simulink model "BallAndPlateSimulation"  (R2019b)
settings: Solver=FixedStepAuto  StartTime=0.0  StopTime=t_experiment  FixedStep=0.001  RelTol=1e-3
values from neighbouring files (symbols this model uses):
  C_v = 16.5    [SimParameters.m]
  g = 9.81    [SimParameters.m]
  I_b = m_b*r_b^2    (= 8.664e-06)    [SimParameters.m]
  I_max = 3    [SimParameters.m]
  I_min = -3    [SimParameters.m]
  I_p = m_p*0.04^2/12    (= 0.00012)    [SimParameters.m]
  K = 11    [SimParameters.m]
  m_b = 0.024    [SimParameters.m]
  m_m = 0.118    [SimParameters.m]
  m_p = 0.9    [SimParameters.m]
  r = 0.17    [SimParameters.m]
  r_b = 0.019    [SimParameters.m]
  Tdelay_bob = 1*10^-9    (= 1e-09)    [SimParameters.m]
  Tdelay_mp = 1*10^-9    (= 1e-09)    [SimParameters.m]
  ts_camera = 1/30    (= 0.0333333333333)    [SimParameters.m]
  ts_mp = 1/1000    (= 0.001)    [SimParameters.m]
  Ybop0 = [0; 0; 0; 0]    [SimParameters.m]
  Ymp0 = [0; 0; 0; 0; 0; Zoffset]    [SimParameters.m]
  Zoffset = 0.32    [SimParameters.m]
undefined symbols (not defined in the file or in its folder): SimulateCamera, SimulateEncoders, SimulateTimeDelays, ts, UseNonlinearPlant
settings Model: Creator=Duintje  LastModifiedBy=chukh

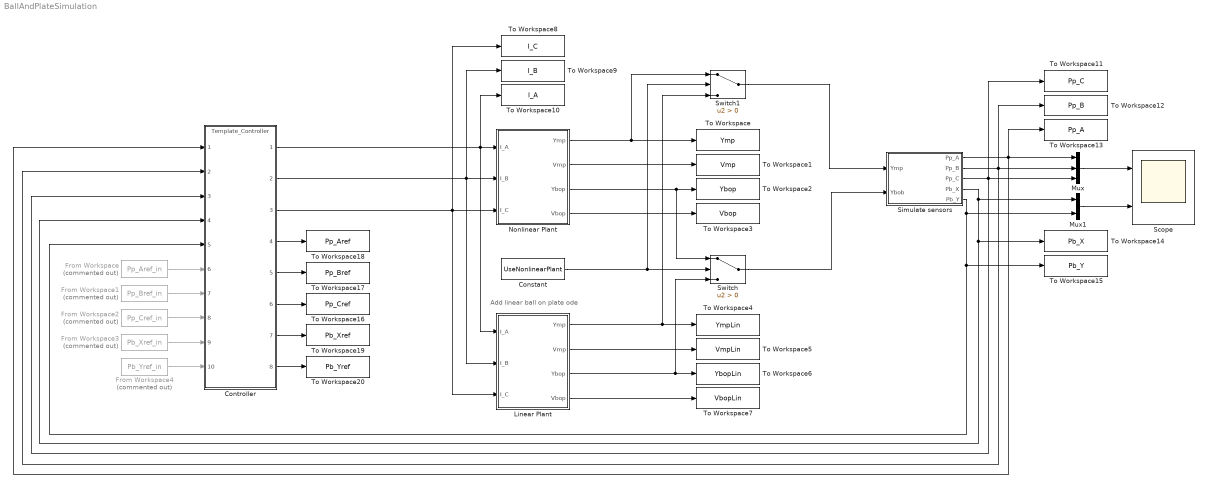
== system BallAndPlateSimulation ==
  note: Add linear ball on plate ode
  Constant : Constant  Value=UseNonlinearPlant
  Controller : ModelReference  ModelNameDialog=Template_Controller.slx  SimulationMode=Normal  ModelReferenceVersion=1.21
  From Workspace : FromWorkspace  Commented=on  VariableName=Pp_Aref_in  SampleTime=ts  Interpolate=off  OutputAfterFinalValue=Holding final value
  From Workspace1 : FromWorkspace  Commented=on  VariableName=Pp_Bref_in  SampleTime=ts  Interpolate=off  OutputAfterFinalValue=Holding final value
  From Workspace2 : FromWorkspace  Commented=on  VariableName=Pp_Cref_in  SampleTime=ts  Interpolate=off  OutputAfterFinalValue=Holding final value
  From Workspace3 : FromWorkspace  Commented=on  VariableName=Pb_Xref_in  SampleTime=ts  Interpolate=off  OutputAfterFinalValue=Holding final value
  From Workspace4 : FromWorkspace  Commented=on  VariableName=Pb_Yref_in  SampleTime=ts  Interpolate=off  OutputAfterFinalValue=Holding final value
  Linear Plant : Subsystem
  Mux : Mux  Inputs=3
  Mux1 : Mux  Inputs=2
  Nonlinear Plant : Subsystem
  Scope : Scope  NumInputPorts=2
  Simulate sensors : Subsystem
  Switch : Switch  Criteria=u2 > Threshold
  Switch1 : Switch  Criteria=u2 > Threshold
  To Workspace : ToWorkspace  VariableName=Ymp  SampleTime=-1
  To Workspace1 : ToWorkspace  VariableName=Vmp  SampleTime=-1
  To Workspace10 : ToWorkspace  VariableName=I_A  SampleTime=-1
  To Workspace11 : ToWorkspace  VariableName=Pp_C  SampleTime=-1
  To Workspace12 : ToWorkspace  VariableName=Pp_B  SampleTime=-1
  To Workspace13 : ToWorkspace  VariableName=Pp_A  SampleTime=-1
  To Workspace14 : ToWorkspace  VariableName=Pb_X  SampleTime=-1
  To Workspace15 : ToWorkspace  VariableName=Pb_Y  SampleTime=-1
  To Workspace16 : ToWorkspace  VariableName=Pp_Cref  SampleTime=-1
  To Workspace17 : ToWorkspace  VariableName=Pp_Bref  SampleTime=-1
  To Workspace18 : ToWorkspace  VariableName=Pp_Aref  SampleTime=-1
  To Workspace19 : ToWorkspace  VariableName=Pb_Xref  SampleTime=-1
  To Workspace2 : ToWorkspace  VariableName=Ybop  SampleTime=-1
  To Workspace20 : ToWorkspace  VariableName=Pb_Yref  SampleTime=-1
  To Workspace3 : ToWorkspace  VariableName=Vbop  SampleTime=-1
  To Workspace4 : ToWorkspace  VariableName=YmpLin  SampleTime=-1
  To Workspace5 : ToWorkspace  VariableName=VmpLin  SampleTime=-1
  To Workspace6 : ToWorkspace  VariableName=YbopLin  SampleTime=-1
  To Workspace7 : ToWorkspace  VariableName=VbopLin  SampleTime=-1
  To Workspace8 : ToWorkspace  VariableName=I_C  SampleTime=-1
  To Workspace9 : ToWorkspace  VariableName=I_B  SampleTime=-1
  wires:
  Controller/1 -> Linear Plant/1(I_A), To Workspace10/1, Nonlinear Plant/1(I_A)
  Controller/2 -> To Workspace9/1, Linear Plant/2(I_B), Nonlinear Plant/2(I_B)
  Controller/3 -> Linear Plant/3(I_C), To Workspace8/1, Nonlinear Plant/3(I_C)
  Linear Plant/1(Ymp) -> Switch1/3, To Workspace4/1
  Linear Plant/2(Vmp) -> To Workspace5/1
  Linear Plant/3(Ybop) -> Switch/3, To Workspace6/1
  Linear Plant/4(Vbop) -> To Workspace7/1
  Nonlinear Plant/3(Ybop) -> Switch/1, To Workspace2/1
  Nonlinear Plant/2(Vmp) -> To Workspace1/1
  Nonlinear Plant/1(Ymp) -> Switch1/1, To Workspace/1
  Nonlinear Plant/4(Vbop) -> To Workspace3/1
  Constant/1 -> Switch1/2, Switch/2
  Switch/1 -> Simulate sensors/2(Ybob)
  Switch1/1 -> Simulate sensors/1(Ymp)
  Simulate sensors/1(Pp_A) -> Controller/1, To Workspace13/1, Mux/1
  Simulate sensors/2(Pp_B) -> Controller/2, To Workspace12/1, Mux/2
  Simulate sensors/3(Pp_C) -> Controller/3, To Workspace11/1, Mux/3
  Mux/1 -> Scope/1
  Simulate sensors/4(Pb_X) -> Mux1/1, Controller/4, To Workspace14/1
  Simulate sensors/5(Pb_Y) -> Mux1/2, Controller/5, To Workspace15/1
  Mux1/1 -> Scope/2
  Controller/4 -> To Workspace18/1
  Controller/5 -> To Workspace17/1
  Controller/6 -> To Workspace16/1
  Controller/7 -> To Workspace19/1
  Controller/8 -> To Workspace20/1
  From Workspace4/1 -> Controller/10
  From Workspace3/1 -> Controller/9
  From Workspace2/1 -> Controller/8
  From Workspace1/1 -> Controller/7
  From Workspace/1 -> Controller/6

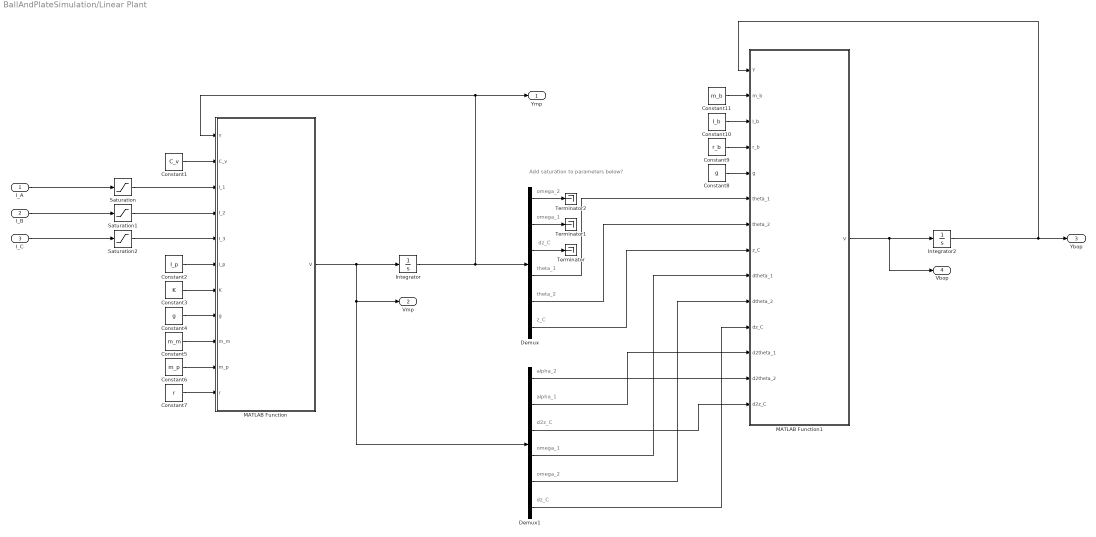
== system BallAndPlateSimulation/Linear Plant ==
  note: Add saturation to parameters below?
  note: omega_2
  note: omega_1
  note: dz_C
  note: theta_1
  note: theta_2
  note: z_C
  note: omega_1
  note: alpha_2
  note: omega_2
  note: alpha_1
  note: dz_C
  note: d2z_C
  I_A : Inport
  I_B : Inport  Port=2
  I_C : Inport  Port=3
  Constant1 : Constant  Value=C_v
  Constant10 : Constant  Value=I_b
  Constant11 : Constant  Value=m_b
  Constant2 : Constant  Value=I_p
  Constant3 : Constant  Value=K
  Constant4 : Constant  Value=g
  Constant5 : Constant  Value=m_m
  Constant6 : Constant  Value=m_p
  Constant7 : Constant  Value=r
  Constant8 : Constant  Value=g
  Constant9 : Constant  Value=r_b
  Demux : Demux  Outputs=6
  Demux1 : Demux  Outputs=6
  Integrator : Integrator  InitialCondition=Ymp0
  Integrator2 : Integrator  InitialCondition=Ybop0
  MATLAB Function : MATLAB Function  TreatAsAtomicUnit=on
  MATLAB Function1 : MATLAB Function  TreatAsAtomicUnit=on
  Saturation : Saturate  UpperLimit=I_max  LowerLimit=I_min
  Saturation1 : Saturate  UpperLimit=I_max  LowerLimit=I_min
  Saturation2 : Saturate  UpperLimit=I_max  LowerLimit=I_min
  Terminator : Terminator
  Terminator1 : Terminator
  Terminator2 : Terminator
  Ymp : Outport
  Vmp : Outport  Port=2
  Ybop : Outport  Port=3
  Vbop : Outport  Port=4
  wires:
  MATLAB Function/1(V) -> Vmp/1, Demux1/1, Integrator/1
  MATLAB Function1/1(V) -> Vbop/1, Integrator2/1
  I_A/1 -> Saturation/1
  Saturation/1 -> MATLAB Function/3(I_1)
  Saturation1/1 -> MATLAB Function/4(I_2)
  Saturation2/1 -> MATLAB Function/5(I_3)
  Constant1/1 -> MATLAB Function/2(C_v)
  Constant2/1 -> MATLAB Function/6(I_p)
  Constant3/1 -> MATLAB Function/7(K)
  Constant4/1 -> MATLAB Function/8(g)
  Constant5/1 -> MATLAB Function/9(m_m)
  Constant6/1 -> MATLAB Function/10(m_p)
  Constant7/1 -> MATLAB Function/11(r)
  Demux1/1 -> MATLAB Function1/13(d2theta_2)
  Demux1/2 -> MATLAB Function1/12(d2theta_1)
  Demux1/6 -> MATLAB Function1/11(dz_C)
  Demux1/3 -> MATLAB Function1/14(d2z_C)
  Demux/6 -> MATLAB Function1/8(z_C)
  Constant8/1 -> MATLAB Function1/5(g)
  Constant9/1 -> MATLAB Function1/4(r_b)
  Constant11/1 -> MATLAB Function1/2(m_b)
  Constant10/1 -> MATLAB Function1/3(I_b)
  Integrator2/1 -> Ybop/1, MATLAB Function1/1(Y)
  I_B/1 -> Saturation1/1
  I_C/1 -> Saturation2/1
  Demux1/4 -> MATLAB Function1/9(dtheta_1)
  Demux1/5 -> MATLAB Function1/10(dtheta_2)
  Demux/5 -> MATLAB Function1/7(theta_2)
  Demux/4 -> MATLAB Function1/6(theta_1)
  Integrator/1 -> Demux/1, Ymp/1, MATLAB Function/1(Y)
  Demux/3 -> Terminator/1
  Demux/2 -> Terminator1/1
  Demux/1 -> Terminator2/1

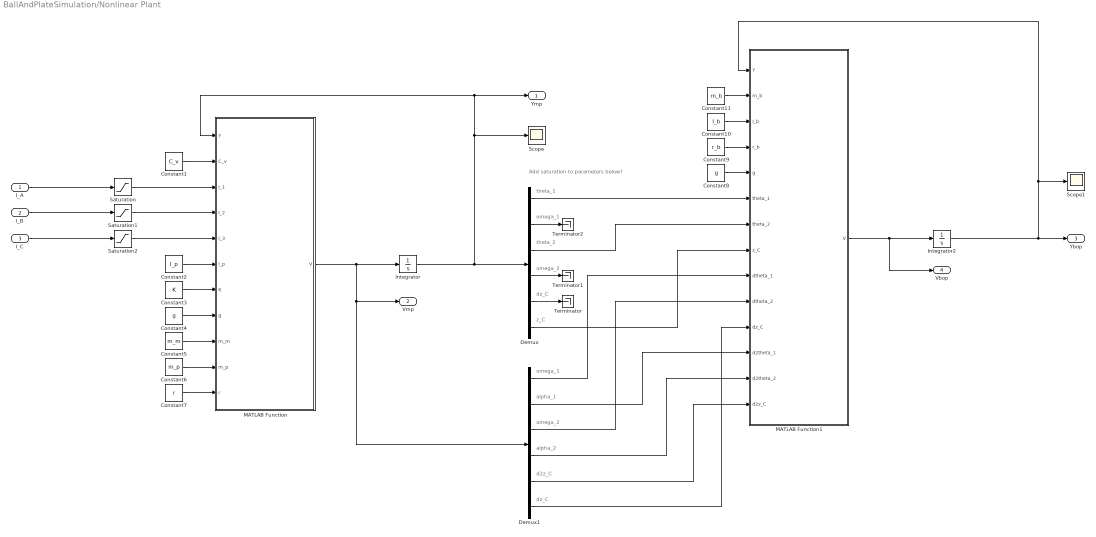
== system BallAndPlateSimulation/Nonlinear Plant ==
  note: Add saturation to parameters below?
  note: theta_1
  note: omega_1
  note: theta_2
  note: omega_2
  note: dz_C
  note: z_C
  note: alpha_2
  note: omega_1
  note: d2z_C
  note: alpha_1
  note: dz_C
  note: omega_2
  I_A : Inport
  I_B : Inport  Port=2
  I_C : Inport  Port=3
  Constant1 : Constant  Value=C_v
  Constant10 : Constant  Value=I_b
  Constant11 : Constant  Value=m_b
  Constant2 : Constant  Value=I_p
  Constant3 : Constant  Value=K
  Constant4 : Constant  Value=g
  Constant5 : Constant  Value=m_m
  Constant6 : Constant  Value=m_p
  Constant7 : Constant  Value=r
  Constant8 : Constant  Value=g
  Constant9 : Constant  Value=r_b
  Demux : Demux  Outputs=6
  Demux1 : Demux  Outputs=6
  Integrator : Integrator  InitialCondition=Ymp0
  Integrator2 : Integrator  InitialCondition=Ybop0
  MATLAB Function : MATLAB Function  TreatAsAtomicUnit=on
  MATLAB Function1 : MATLAB Function  TreatAsAtomicUnit=on
  Saturation : Saturate  UpperLimit=I_max  LowerLimit=I_min
  Saturation1 : Saturate  UpperLimit=I_max  LowerLimit=I_min
  Saturation2 : Saturate  UpperLimit=I_max  LowerLimit=I_min
  Scope : Scope
  Scope1 : Scope
  Terminator : Terminator
  Terminator1 : Terminator
  Terminator2 : Terminator
  Ymp : Outport
  Vmp : Outport  Port=2
  Ybop : Outport  Port=3
  Vbop : Outport  Port=4
  wires:
  MATLAB Function/1(V) -> Vmp/1, Demux1/1, Integrator/1
  MATLAB Function1/1(V) -> Vbop/1, Integrator2/1
  I_A/1 -> Saturation/1
  Saturation/1 -> MATLAB Function/3(I_1)
  Saturation1/1 -> MATLAB Function/4(I_2)
  Saturation2/1 -> MATLAB Function/5(I_3)
  Constant1/1 -> MATLAB Function/2(C_v)
  Constant2/1 -> MATLAB Function/6(I_p)
  Constant3/1 -> MATLAB Function/7(K)
  Constant4/1 -> MATLAB Function/8(g)
  Constant5/1 -> MATLAB Function/9(m_m)
  Constant6/1 -> MATLAB Function/10(m_p)
  Constant7/1 -> MATLAB Function/11(r)
  Integrator/1 -> Demux/1, Ymp/1, MATLAB Function/1(Y), Scope/1
  Demux/1 -> MATLAB Function1/6(theta_1)
  Demux1/1 -> MATLAB Function1/9(dtheta_1)
  Demux1/5 -> MATLAB Function1/14(d2z_C)
  Demux1/4 -> MATLAB Function1/13(d2theta_2)
  Demux1/2 -> MATLAB Function1/12(d2theta_1)
  Demux1/6 -> MATLAB Function1/11(dz_C)
  Demux1/3 -> MATLAB Function1/10(dtheta_2)
  Demux/6 -> MATLAB Function1/8(z_C)
  Demux/3 -> MATLAB Function1/7(theta_2)
  Constant8/1 -> MATLAB Function1/5(g)
  Constant9/1 -> MATLAB Function1/4(r_b)
  Constant11/1 -> MATLAB Function1/2(m_b)
  Constant10/1 -> MATLAB Function1/3(I_b)
  Integrator2/1 -> Ybop/1, Scope1/1, MATLAB Function1/1(Y)
  I_B/1 -> Saturation1/1
  I_C/1 -> Saturation2/1
  Demux/5 -> Terminator/1
  Demux/4 -> Terminator1/1
  Demux/2 -> Terminator2/1

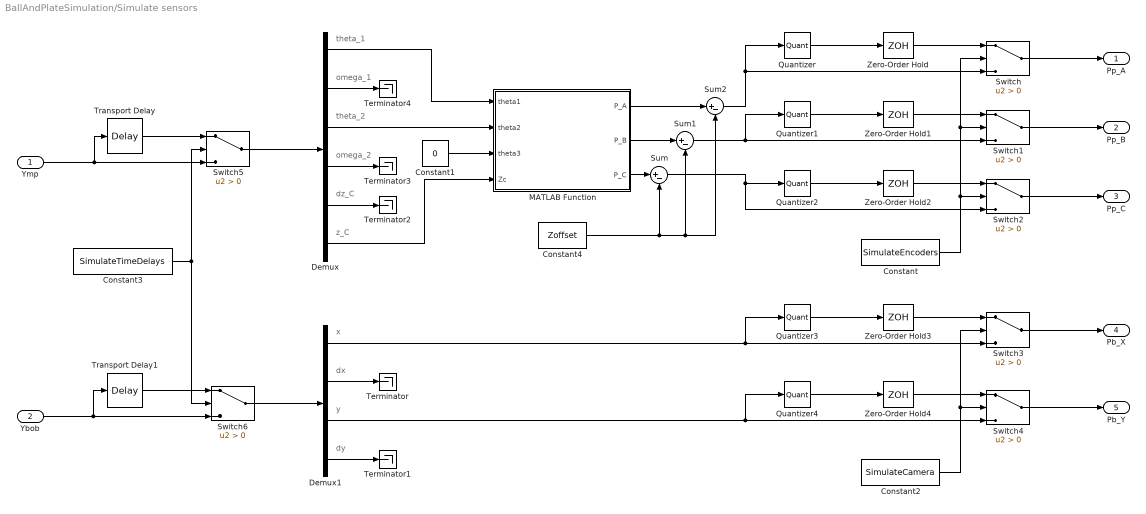
== system BallAndPlateSimulation/Simulate sensors ==
  note: dx
  note: dy
  note: x
  note: y
  note: theta_1
  note: omega_2
  note: dz_C
  note: theta_2
  note: z_C
  note: omega_1
  Ymp : Inport
  Ybob : Inport  Port=2
  Constant : Constant  Value=SimulateEncoders
  Constant1 : Constant  Value=0
  Constant2 : Constant  Value=SimulateCamera
  Constant3 : Constant  Value=SimulateTimeDelays
  Constant4 : Constant  Value=Zoffset
  Demux : Demux  Outputs=6
  Demux1 : Demux
  MATLAB Function : MATLAB Function  TreatAsAtomicUnit=on
  Quantizer : Quantizer  QuantizationInterval=EncStepSize
  Quantizer1 : Quantizer  QuantizationInterval=EncStepSize
  Quantizer2 : Quantizer  QuantizationInterval=EncStepSize
  Quantizer3 : Quantizer  QuantizationInterval=CameraStepSize
  Quantizer4 : Quantizer  QuantizationInterval=CameraStepSize
  Sum : Sum  Inputs=|+-
  Sum1 : Sum  Inputs=|+-
  Sum2 : Sum  Inputs=|+-
  Switch{,1..6} (7 alike) : Switch  Criteria=u2 > Threshold
  Terminator{,1..4} (5 alike) : Terminator
  Transport Delay : TransportDelay  DelayTime=Tdelay_mp
  Transport Delay1 : TransportDelay  DelayTime=Tdelay_bob
  Zero-Order Hold : ZeroOrderHold  SampleTime=ts_mp
  Zero-Order Hold1 : ZeroOrderHold  SampleTime=ts_mp
  Zero-Order Hold2 : ZeroOrderHold  SampleTime=ts_mp
  Zero-Order Hold3 : ZeroOrderHold  SampleTime=ts_camera
  Zero-Order Hold4 : ZeroOrderHold  SampleTime=ts_camera
  Pp_A : Outport
  Pp_B : Outport  Port=2
  Pp_C : Outport  Port=3
  Pb_X : Outport  Port=4
  Pb_Y : Outport  Port=5
  wires:
  Demux/3 -> MATLAB Function/2(theta2)
  Demux/6 -> MATLAB Function/4(Zc)
  Demux/1 -> MATLAB Function/1(theta1)
  Ymp/1 -> Transport Delay/1, Switch5/3
  Constant1/1 -> MATLAB Function/3(theta3)
  Sum2/1 -> Quantizer/1, Switch/3
  Zero-Order Hold/1 -> Switch/1
  Quantizer/1 -> Zero-Order Hold/1
  Switch/1 -> Pp_A/1
  Quantizer1/1 -> Zero-Order Hold1/1
  Switch1/1 -> Pp_B/1
  Zero-Order Hold1/1 -> Switch1/1
  Sum1/1 -> Quantizer1/1, Switch1/3
  Quantizer2/1 -> Zero-Order Hold2/1
  Switch2/1 -> Pp_C/1
  Zero-Order Hold2/1 -> Switch2/1
  Sum/1 -> Quantizer2/1, Switch2/3
  Constant/1 -> Switch2/2, Switch/2, Switch1/2
  Zero-Order Hold3/1 -> Switch3/1
  Quantizer3/1 -> Zero-Order Hold3/1
  Zero-Order Hold4/1 -> Switch4/1
  Demux1/3 -> Quantizer4/1, Switch4/3
  Constant2/1 -> Switch3/2, Switch4/2
  Switch4/1 -> Pb_Y/1
  Demux1/1 -> Quantizer3/1, Switch3/3
  Quantizer4/1 -> Zero-Order Hold4/1
  Switch3/1 -> Pb_X/1
  Switch5/1 -> Demux/1
  Transport Delay/1 -> Switch5/1
  Ybob/1 -> Switch6/3, Transport Delay1/1
  Switch6/1 -> Demux1/1
  Transport Delay1/1 -> Switch6/1
  Constant3/1 -> Switch5/2, Switch6/2
  MATLAB Function/3(P_C) -> Sum/1
  MATLAB Function/2(P_B) -> Sum1/1
  MATLAB Function/1(P_A) -> Sum2/1
  Constant4/1 -> Sum2/2, Sum1/2, Sum/2
  Demux1/2 -> Terminator/1
  Demux1/4 -> Terminator1/1
  Demux/5 -> Terminator2/1
  Demux/4 -> Terminator3/1
  Demux/2 -> Terminator4/1

== matlab function BallAndPlateSimulation/Nonlinear Plant/MATLAB Function1 ==
  data: Y input; V output; m_b input; I_b input; r_b input; g input; theta_1 input; theta_2 input; z_C input; dtheta_1 input; dtheta_2 input; dz_C input; d2theta_1 input; d2theta_2 input; d2z_C input
function V = ballOnPlateODE(Y,m_b,I_b,r_b,g,theta_1,theta_2,z_C,dtheta_1,dtheta_2,dz_C,d2theta_1,d2theta_2,d2z_C)
%BALLONPLATEODE
%    V = BALLONPLATEODE(Y,M_B,I_B,R_B,G,THETA_1,THETA_2,Z_C,DTHETA_1,DTHETA_2,DZ_C,D2THETA_1,D2THETA_2,D2Z_C)

%    This function was generated by the Symbolic Math Toolbox version 8.4.
%    26-May-2021 19:55:45

%matrix([[xf], [Dxf], [yf], [Dyf]])
t2 = cos(theta_1);
t3 = cos(theta_2);
t4 = sin(theta_1);
t5 = sin(theta_2);
t6 = Y(1);
t7 = Y(2);
t8 = Y(3);
t9 = Y(4);
t10 = dtheta_1.^2;
t11 = dtheta_2.^2;
t12 = r_b.^2;
t13 = r_b.^3;
t14 = t2.^2;
t15 = t2.^3;
t16 = t3.^2;
t18 = t3.^3;
t20 = t4.^2;
t21 = t4.^3;
t22 = t5.^2;
t24 = t5.^3;
t28 = m_b.*t12;
t17 = t14.^2;
t19 = t16.^2;
t23 = t20.^2;
t25 = t22.^2;
t26 = 1.0./t14;
t27 = 1.0./t16;
t29 = I_b+t28;
t30 = t14+t20;
t31 = 1.0./t29;
t32 = 1.0./t30;
V = [t7;(t26.*t27.*t31.*t32.*(I_b.*d2theta_2.*r_b.*t15.*t18+I_b.*r_b.*t11.*t15.*t24.*2.0-I_b.*t6.*t11.*t17.*t19-I_b.*t6.*t11.*t17.*t25.*2.0+d2z_C.*t5.*t17.*t18.*t28+g.*t5.*t17.*t18.*t28+m_b.*t11.*t13.*t15.*t24.*2.0-t6.*t11.*t17.*t25.*t28.*2.0+d2theta_2.*m_b.*t3.*t13.*t15.*t22+d2theta_1.*t5.*t8.*t16.*t17.*t28-d2theta_2.*t5.*t6.*t17.*t18.*t28-d2theta_2.*t3.*t6.*t17.*t24.*t28+dtheta_1.*t5.*t9.*t16.*t17.*t28.*2.0-dtheta_2.*t5.*t7.*t17.*t18.*t28.*2.0+dtheta_1.*t5.*t9.*t17.*t18.*t28-dtheta_2.*t3.*t7.*t17.*t24.*t28.*2.0+m_b.*t5.*t10.*t13.*t15.*t16.*2.0+m_b.*t5.*t11.*t13.*t15.*t16+t4.*t8.*t11.*t15.*t24.*t28.*2.0-t6.*t10.*t16.*t17.*t22.*t28-t6.*t11.*t16.*t17.*t22.*t28.*2.0+I_b.*dtheta_1.*dtheta_2.*r_b.*t18.*t21.*2.0+I_b.*dtheta_1.*dtheta_2.*t8.*t17.*t18.*2.0-I_b.*dtheta_1.*dtheta_2.*t8.*t17.*t19+I_b.*dtheta_1.*dtheta_2.*t8.*t18.*t23.*2.0+I_b.*d2theta_2.*r_b.*t2.*t18.*t20+I_b.*d2theta_2.*r_b.*t3.*t15.*t22+I_b.*d2theta_1.*t5.*t8.*t16.*t17+I_b.*d2theta_2.*t4.*t8.*t15.*t18-I_b.*d2theta_2.*t5.*t6.*t17.*t18-I_b.*d2theta_1.*t5.*t8.*t17.*t18+I_b.*d2theta_2.*t2.*t8.*t18.*t21-I_b.*d2theta_2.*t3.*t6.*t17.*t24+I_b.*dtheta_1.*t5.*t9.*t16.*t17.*2.0+I_b.*dtheta_2.*t4.*t9.*t15.*t18.*2.0-I_b.*dtheta_2.*t5.*t7.*t17.*t18.*2.0-I_b.*dtheta_1.*t5.*t9.*t17.*t18+I_b.*dtheta_2.*t2.*t9.*t18.*t21.*2.0-I_b.*dtheta_2.*t3.*t7.*t17.*t24.*2.0+I_b.*r_b.*t5.*t10.*t15.*t16+I_b.*r_b.*t5.*t11.*t15.*t16.*2.0+I_b.*r_b.*t2.*t11.*t20.*t24.*2.0+I_b.*t4.*t8.*t11.*t15.*t24.*2.0+I_b.*t2.*t8.*t11.*t21.*t24.*2.0-I_b.*t6.*t11.*t14.*t19.*t20-I_b.*t6.*t11.*t16.*t17.*t22.*3.0-I_b.*t6.*t11.*t14.*t20.*t25.*2.0+I_b.*dtheta_1.*dtheta_2.*r_b.*t4.*t14.*t18.*2.0-I_b.*dtheta_1.*dtheta_2.*r_b.*t4.*t14.*t22+I_b.*dtheta_1.*dtheta_2.*r_b.*t3.*t21.*t22.*2.0+I_b.*dtheta_1.*dtheta_2.*t4.*t6.*t15.*t24+I_b.*dtheta_1.*dtheta_2.*t3.*t8.*t17.*t22.*2.0+I_b.*dtheta_1.*dtheta_2.*t3.*t8.*t22.*t23.*2.0+I_b.*dtheta_1.*dtheta_2.*t8.*t14.*t18.*t20.*4.0-I_b.*dtheta_1.*dtheta_2.*t8.*t14.*t19.*t20-I_b.*dtheta_1.*dtheta_2.*t8.*t14.*t20.*t22-I_b.*d2theta_1.*r_b.*t3.*t4.*t5.*t14+I_b.*d2theta_1.*r_b.*t4.*t5.*t14.*t16+I_b.*d2theta_2.*r_b.*t2.*t3.*t20.*t22+I_b.*d2theta_1.*t3.*t4.*t6.*t15.*t22-I_b.*d2theta_1.*t3.*t5.*t8.*t14.*t20+I_b.*d2theta_2.*t3.*t4.*t8.*t15.*t22+I_b.*d2theta_2.*t2.*t3.*t8.*t21.*t22+I_b.*d2theta_1.*t5.*t8.*t14.*t16.*t20-I_b.*d2theta_2.*t5.*t6.*t14.*t18.*t20-I_b.*d2theta_2.*t3.*t6.*t14.*t20.*t24+I_b.*dtheta_1.*t3.*t4.*t7.*t15.*t22-I_b.*dtheta_1.*t3.*t5.*t9.*t14.*t20+I_b.*dtheta_2.*t3.*t4.*t9.*t15.*t22.*2.0+I_b.*dtheta_2.*t2.*t3.*t9.*t21.*t22.*2.0+I_b.*dtheta_1.*t5.*t9.*t14.*t16.*t20.*2.0-I_b.*dtheta_2.*t5.*t7.*t14.*t18.*t20.*2.0-I_b.*dtheta_2.*t3.*t7.*t14.*t20.*t24.*2.0+I_b.*r_b.*t2.*t5.*t10.*t16.*t20+I_b.*r_b.*t2.*t5.*t11.*t16.*t20.*2.0-I_b.*t3.*t4.*t5.*t8.*t10.*t15+I_b.*t4.*t5.*t8.*t10.*t15.*t16+I_b.*t4.*t5.*t8.*t11.*t15.*t16.*2.0+I_b.*t4.*t5.*t8.*t10.*t15.*t18+I_b.*t2.*t5.*t8.*t10.*t16.*t21+I_b.*t2.*t5.*t8.*t11.*t16.*t21.*2.0-I_b.*t3.*t6.*t10.*t14.*t20.*t22-I_b.*t6.*t11.*t14.*t16.*t20.*t22.*3.0+dtheta_1.*dtheta_2.*m_b.*t4.*t13.*t14.*t22-dtheta_1.*dtheta_2.*t4.*t6.*t15.*t24.*t28+dtheta_1.*dtheta_2.*t3.*t8.*t17.*t22.*t28.*2.0+dtheta_1.*dtheta_2.*t8.*t14.*t20.*t22.*t28+d2theta_1.*m_b.*t4.*t5.*t13.*t14.*t16+d2theta_2.*t3.*t4.*t8.*t15.*t22.*t28+d2theta_1.*t5.*t8.*t14.*t16.*t20.*t28-dtheta_1.*t3.*t4.*t7.*t15.*t22.*t28+dtheta_1.*t3.*t5.*t9.*t14.*t20.*t28+dtheta_2.*t3.*t4.*t9.*t15.*t22.*t28.*2.0+dtheta_1.*t5.*t9.*t14.*t16.*t20.*t28.*2.0+m_b.*t2.*t3.*t5.*t10.*t13.*t20.*2.0+m_b.*t2.*t5.*t10.*t13.*t16.*t20+t3.*t4.*t5.*t8.*t10.*t15.*t28+t2.*t3.*t5.*t8.*t10.*t21.*t28.*2.0+t4.*t5.*t8.*t10.*t15.*t16.*t28+t4.*t5.*t8.*t11.*t15.*t16.*t28+t4.*t5.*t8.*t10.*t15.*t18.*t28+t2.*t5.*t8.*t10.*t16.*t21.*t28-t3.*t6.*t10.*t14.*t20.*t22.*t28+I_b.*dtheta_1.*dtheta_2.*r_b.*t3.*t4.*t14.*t22.*2.0+I_b.*dtheta_1.*dtheta_2.*t4.*t5.*t6.*t15.*t16+I_b.*dtheta_1.*dtheta_2.*t3.*t8.*t14.*t20.*t22.*4.0-I_b.*dtheta_1.*dtheta_2.*t8.*t14.*t16.*t20.*t22+dtheta_1.*dtheta_2.*m_b.*t3.*t4.*t13.*t14.*t22.*2.0+dtheta_1.*dtheta_2.*t3.*t8.*t14.*t20.*t22.*t28.*2.0))./(t16+t22);t9;-t26.*t27.*t31.*t32.*(I_b.*d2theta_1.*r_b.*t3.*t15+I_b.*r_b.*t10.*t16.*t21.*2.0+I_b.*t3.*t8.*t10.*t17+I_b.*t8.*t10.*t16.*t17-I_b.*t8.*t10.*t17.*t18+I_b.*t8.*t10.*t16.*t23.*2.0+d2z_C.*t4.*t15.*t18.*t28+g.*t4.*t15.*t18.*t28+m_b.*t10.*t13.*t16.*t21.*2.0-t3.*t8.*t10.*t17.*t28+t8.*t10.*t16.*t17.*t28.*2.0-t8.*t10.*t17.*t18.*t28+t8.*t10.*t16.*t23.*t28.*2.0+d2theta_1.*m_b.*t2.*t13.*t16.*t20+d2theta_1.*t4.*t8.*t15.*t16.*t28-d2theta_2.*t4.*t6.*t15.*t18.*t28+d2theta_1.*t2.*t8.*t16.*t21.*t28-dtheta_1.*t3.*t4.*t9.*t15.*t28+dtheta_1.*t3.*t5.*t7.*t17.*t28+dtheta_1.*t4.*t9.*t15.*t16.*t28.*2.0-dtheta_2.*t4.*t7.*t15.*t18.*t28.*2.0+dtheta_1.*t4.*t9.*t15.*t18.*t28+dtheta_1.*t2.*t9.*t16.*t21.*t28.*2.0-m_b.*t3.*t4.*t10.*t13.*t14.*2.0+m_b.*t4.*t10.*t13.*t14.*t16.*3.0+m_b.*t4.*t11.*t13.*t14.*t16+m_b.*t4.*t11.*t13.*t14.*t22.*2.0-t3.*t8.*t10.*t14.*t20.*t28.*2.0-t4.*t6.*t11.*t15.*t24.*t28.*2.0+t8.*t10.*t14.*t16.*t20.*t28.*4.0+t8.*t11.*t14.*t16.*t20.*t28+t8.*t11.*t14.*t20.*t22.*t28.*2.0+I_b.*dtheta_1.*dtheta_2.*r_b.*t5.*t15-I_b.*dtheta_1.*dtheta_2.*t6.*t16.*t17-I_b.*dtheta_1.*dtheta_2.*t6.*t17.*t22+I_b.*d2theta_1.*r_b.*t2.*t16.*t20+I_b.*d2theta_1.*t3.*t4.*t8.*t15-I_b.*d2theta_1.*t3.*t5.*t6.*t17+I_b.*d2theta_1.*t4.*t8.*t15.*t16-I_b.*d2theta_1.*t4.*t8.*t15.*t18+I_b.*d2theta_1.*t2.*t8.*t16.*t21+I_b.*dtheta_1.*t3.*t4.*t9.*t15-I_b.*dtheta_1.*t3.*t5.*t7.*t17+I_b.*dtheta_1.*t4.*t9.*t15.*t16.*2.0-I_b.*dtheta_1.*t4.*t9.*t15.*t18+I_b.*dtheta_1.*t2.*t9.*t16.*t21.*2.0+I_b.*r_b.*t4.*t10.*t14.*t16.*2.0+I_b.*t8.*t10.*t14.*t16.*t20.*3.0-dtheta_1.*dtheta_2.*m_b.*t5.*t13.*t15+dtheta_1.*dtheta_2.*t6.*t17.*t22.*t28+I_b.*dtheta_1.*dtheta_2.*t4.*t5.*t8.*t15+I_b.*t3.*t4.*t5.*t6.*t10.*t15-dtheta_1.*dtheta_2.*t4.*t5.*t8.*t15.*t28+d2theta_2.*m_b.*t3.*t4.*t5.*t13.*t14-d2theta_2.*t3.*t4.*t6.*t15.*t22.*t28+d2theta_2.*t3.*t5.*t8.*t14.*t20.*t28-dtheta_2.*t3.*t4.*t7.*t15.*t22.*t28.*2.0+dtheta_2.*t3.*t5.*t9.*t14.*t20.*t28.*2.0+t3.*t4.*t5.*t6.*t10.*t15.*t28-t4.*t5.*t6.*t10.*t15.*t16.*t28-t4.*t5.*t6.*t11.*t15.*t16.*t28.*2.0+I_b.*dtheta_1.*dtheta_2.*t4.*t5.*t8.*t15.*t16+dtheta_1.*dtheta_2.*m_b.*t2.*t3.*t5.*t13.*t20.*2.0+dtheta_1.*dtheta_2.*t3.*t4.*t5.*t8.*t15.*t28.*2.0+dtheta_1.*dtheta_2.*t2.*t3.*t5.*t8.*t21.*t28.*2.0)];

== matlab function BallAndPlateSimulation/Nonlinear Plant/MATLAB Function ==
  data: Y input; V output; C_v input; I_1 input; I_2 input; I_3 input; I_p input; K input; g input; m_m input; m_p input; r input
function V = motorPlateODE(Y,C_v,I_1,I_2,I_3,I_p,K,g,m_m,m_p,r)
%MOTORPLATEODE
%    V = MOTORPLATEODE(Y,C_v,I_1,I_2,I_3,I_p,K,g,m_m,m_p,r)

%    This function was generated by the Symbolic Math Toolbox version 8.4.
%    18-May-2021 19:45:09

%matrix([[theta_1f], [omega_1f], [theta_2f], [omega_2f], [dz_Cf], [z_Cf]])
t2 = I_p.^2;
t3 = Y(1);
t4 = Y(2);
t5 = Y(3);
t6 = Y(4);
t7 = Y(5);
t8 = m_m.^2;
t9 = r.^2;
t10 = r.^3;
t19 = sqrt(3.0);
t11 = t9.^2;
t12 = cos(t3);
t13 = cos(t5);
t14 = sin(t3);
t15 = sin(t5);
t16 = t2.*4.0;
t17 = t4.^2;
t18 = t6.^2;
t20 = t12.^2;
t21 = t12.^3;
t22 = t13.^2;
t23 = t13.^3;
t25 = t14.^2;
t26 = t15.^2;
t24 = t22.^2;
t27 = I_p.*m_m.*t9.*t22.*6.0;
t29 = I_p.*m_m.*t9.*t25.*t26.*6.0;
t28 = t20.*t27;
t30 = t8.*t11.*t20.*t24.*9.0;
t31 = t16+t27+t28+t29+t30;
t32 = 1.0./t31;
V = [t4;t32.*(t12.*t14.*t17.*t27+t12.*t14.*t18.*t27+t8.*t11.*t12.*t14.*t17.*t24.*9.0+t8.*t11.*t12.*t14.*t18.*t24.*9.0-C_v.*I_p.*t4.*t9.*t20.*t22.*6.0-C_v.*m_m.*t4.*t11.*t20.*t24.*9.0+I_2.*I_p.*K.*r.*t12.*t13.*t19.*2.0-I_3.*I_p.*K.*r.*t12.*t13.*t19.*2.0+I_2.*K.*m_m.*t10.*t12.*t19.*t23.*3.0-I_3.*K.*m_m.*t10.*t12.*t19.*t23.*3.0+t4.*t6.*t8.*t11.*t15.*t20.*t23.*1.8e+1+t8.*t11.*t12.*t14.*t18.*t22.*t26.*1.8e+1-t8.*t11.*t14.*t18.*t21.*t22.*t26.*9.0-t8.*t11.*t12.*t14.^3.*t18.*t22.*t26.*9.0-t4.*t6.*t8.*t11.*t13.*t15.^3.*t20.*t25.*9.0+C_v.*I_p.*t6.*t9.*t12.*t13.*t14.*t15.*6.0-I_1.*K.*m_m.*t10.*t12.*t14.*t15.*t22.*6.0+I_2.*K.*m_m.*t10.*t12.*t14.*t15.*t22.*3.0+I_3.*K.*m_m.*t10.*t12.*t14.*t15.*t22.*3.0+I_p.*m_m.*t4.*t6.*t9.*t13.*t15.*t20.*1.2e+1+t4.*t6.*t8.*t11.*t13.*t15.*t20.*t25.*9.0-t4.*t6.*t8.*t11.*t15.*t20.*t23.*t25.*9.0);t6;-r.*t32.*(I_1.*I_p.*K.*t13.*4.0-I_2.*I_p.*K.*t13.*2.0-I_3.*I_p.*K.*t13.*2.0+C_v.*I_p.*r.*t6.*t22.*6.0-t8.*t10.*t15.*t18.*t20.*t23.*1.8e+1+t8.*t10.*t15.*t18.*t20.^2.*t23.*9.0+I_2.*I_p.*K.*t14.*t15.*t19.*2.0-I_3.*I_p.*K.*t14.*t15.*t19.*2.0+C_v.*I_p.*r.*t6.*t25.*t26.*6.0+I_1.*K.*m_m.*t9.*t20.*t23.*6.0-I_2.*K.*m_m.*t9.*t20.*t23.*3.0-I_3.*K.*m_m.*t9.*t20.*t23.*3.0+C_v.*m_m.*t6.*t10.*t20.*t24.*9.0-I_p.*m_m.*r.*t13.*t15.*t18.*1.2e+1-I_p.*m_m.*r.*t4.*t6.*t12.*t14.*6.0+I_p.*m_m.*r.*t13.*t15.*t18.*t20.*6.0+I_p.*m_m.*r.*t13.*t15.*t17.*t25.*6.0+I_p.*m_m.*r.*t13.*t15.*t18.*t25.*1.2e+1-t4.*t6.*t8.*t10.*t14.*t21.*t22.*9.0+t4.*t6.*t8.*t10.*t14.*t21.*t24.*9.0+t8.*t10.*t15.*t18.*t20.*t23.*t25.*9.0-C_v.*I_p.*r.*t4.*t12.*t13.*t14.*t15.*6.0+I_p.*m_m.*r.*t4.*t6.*t12.*t14.*t22.*6.0+I_p.*m_m.*r.*t4.*t6.*t12.*t14.*t26.*1.8e+1+t4.*t6.*t8.*t10.*t14.*t21.*t22.*t26.*9.0);-(C_v.*t7.*3.0+g.*m_m.*3.0+g.*m_p-I_1.*K-I_2.*K-I_3.*K)./(m_m.*3.0+m_p);t7];
end

== matlab function BallAndPlateSimulation/Linear Plant/MATLAB Function ==
  data: Y input; V output; C_v input; I_1 input; I_2 input; I_3 input; I_p input; K input; g input; m_m input; m_p input; r input
function V = motorPlateODElinear(Y,C_v,I_1,I_2,I_3,I_p,K,g,m_m,m_p,r)
%MOTORPLATEODELINEAR
%    V = MOTORPLATEODELINEAR(Y,C_v,I_1,I_2,I_3,I_p,K,g,m_m,m_p,r)

%    This function was generated by the Symbolic Math Toolbox version 58.4.
%    13-May-2021 20:04:38

%matrix([[omega_2f], [omega_1f], [dz_Cf], [theta_1f], [theta_2f], [z_Cf]])
t2 = I_p.*2.0;
t3 = Y(1);
t4 = Y(2);
t5 = Y(3);
t6 = r.^2;
t7 = I_2.*K;
t8 = I_3.*K;
t9 = sqrt(3.0);
t10 = -t7;
t11 = -t8;
t12 = m_m.*t6.*3.0;
t13 = t2+t12;
t14 = 1.0./t13;
V = [r.*t14.*(t7+t8-I_1.*K.*2.0-C_v.*r.*t3.*3.0);-r.*t14.*(t8.*t9+t9.*t10+C_v.*r.*t4.*3.0);-(m_p+t10+t11+C_v.*t5.*3.0+g.*m_m.*3.0-I_1.*K)./(m_m.*3.0+m_p);t4;t3;t5];
end

== matlab function BallAndPlateSimulation/Linear Plant/MATLAB Function1 ==
  data: Y input; V output; m_b input; I_b input; r_b input; g input; theta_1 input; theta_2 input; z_C input; dtheta_1 input; dtheta_2 input; dz_C input; d2theta_1 input; d2theta_2 input; d2z_C input
function V = ballOnPlateODE(Y,m_b,I_b,r_b,g,theta_1,theta_2,z_C,dtheta_1,dtheta_2,dz_C,d2theta_1,d2theta_2,d2z_C)
%BALLONPLATEODE
%    V = BALLONPLATEODE(Y,m_b,I_b,r_b,g,theta_1,theta_2,z_C,dtheta_1,dtheta_2,dz_C,d2theta_1,d2theta_2,d2z_C)

%    This function was generated by the Symbolic Math Toolbox version 8.4.
%    16-May-2021 00:03:52

%matrix([[xf], [Dxf], [yf], [Dyf]])
t2 = cos(theta_1);
t3 = cos(theta_2);
t4 = sin(theta_1);
t5 = sin(theta_2);
t6 = Y(1);
t7 = Y(2);
t8 = Y(3);
t9 = Y(4);
t10 = dtheta_1.^2;
t11 = dtheta_2.^2;
t12 = r_b.^2;
t13 = r_b.^3;
t14 = t2.^2;
t15 = t2.^3;
t16 = t3.^2;
t18 = t3.^3;
t20 = t4.^2;
t21 = t4.^3;
t22 = t5.^2;
t24 = t5.^3;
t28 = m_b.*t12;
t17 = t14.^2;
t19 = t16.^2;
t23 = t20.^2;
t25 = t22.^2;
t26 = 1.0./t14;
t27 = 1.0./t16;
t29 = I_b+t28;
t30 = t14+t20;
t31 = 1.0./t29;
t32 = 1.0./t30;
V = [t7;(t26.*t27.*t31.*t32.*(I_b.*d2theta_2.*r_b.*t15.*t18+I_b.*r_b.*t11.*t15.*t24.*2.0-I_b.*t6.*t11.*t17.*t19-I_b.*t6.*t11.*t17.*t25.*2.0+d2z_C.*t5.*t17.*t18.*t28+g.*t5.*t17.*t18.*t28+m_b.*t11.*t13.*t15.*t24.*2.0-t6.*t11.*t17.*t25.*t28.*2.0+d2theta_2.*m_b.*t3.*t13.*t15.*t22+d2theta_1.*t5.*t8.*t16.*t17.*t28-d2theta_2.*t5.*t6.*t17.*t18.*t28-d2theta_2.*t3.*t6.*t17.*t24.*t28+dtheta_1.*t5.*t9.*t16.*t17.*t28.*2.0-dtheta_2.*t5.*t7.*t17.*t18.*t28.*2.0+dtheta_1.*t5.*t9.*t17.*t18.*t28-dtheta_2.*t3.*t7.*t17.*t24.*t28.*2.0+m_b.*t5.*t10.*t13.*t15.*t16.*2.0+m_b.*t5.*t11.*t13.*t15.*t16+t4.*t8.*t11.*t15.*t24.*t28.*2.0-t6.*t10.*t16.*t17.*t22.*t28-t6.*t11.*t16.*t17.*t22.*t28.*2.0+I_b.*dtheta_1.*dtheta_2.*r_b.*t18.*t21.*2.0+I_b.*dtheta_1.*dtheta_2.*t8.*t17.*t18.*2.0-I_b.*dtheta_1.*dtheta_2.*t8.*t17.*t19+I_b.*dtheta_1.*dtheta_2.*t8.*t18.*t23.*2.0+I_b.*d2theta_2.*r_b.*t2.*t18.*t20+I_b.*d2theta_2.*r_b.*t3.*t15.*t22+I_b.*d2theta_1.*t5.*t8.*t16.*t17+I_b.*d2theta_2.*t4.*t8.*t15.*t18-I_b.*d2theta_2.*t5.*t6.*t17.*t18-I_b.*d2theta_1.*t5.*t8.*t17.*t18+I_b.*d2theta_2.*t2.*t8.*t18.*t21-I_b.*d2theta_2.*t3.*t6.*t17.*t24+I_b.*dtheta_1.*t5.*t9.*t16.*t17.*2.0+I_b.*dtheta_2.*t4.*t9.*t15.*t18.*2.0-I_b.*dtheta_2.*t5.*t7.*t17.*t18.*2.0-I_b.*dtheta_1.*t5.*t9.*t17.*t18+I_b.*dtheta_2.*t2.*t9.*t18.*t21.*2.0-I_b.*dtheta_2.*t3.*t7.*t17.*t24.*2.0+I_b.*r_b.*t5.*t10.*t15.*t16+I_b.*r_b.*t5.*t11.*t15.*t16.*2.0+I_b.*r_b.*t2.*t11.*t20.*t24.*2.0+I_b.*t4.*t8.*t11.*t15.*t24.*2.0+I_b.*t2.*t8.*t11.*t21.*t24.*2.0-I_b.*t6.*t11.*t14.*t19.*t20-I_b.*t6.*t11.*t16.*t17.*t22.*3.0-I_b.*t6.*t11.*t14.*t20.*t25.*2.0+I_b.*dtheta_1.*dtheta_2.*r_b.*t4.*t14.*t18.*2.0-I_b.*dtheta_1.*dtheta_2.*r_b.*t4.*t14.*t22+I_b.*dtheta_1.*dtheta_2.*r_b.*t3.*t21.*t22.*2.0+I_b.*dtheta_1.*dtheta_2.*t4.*t6.*t15.*t24+I_b.*dtheta_1.*dtheta_2.*t3.*t8.*t17.*t22.*2.0+I_b.*dtheta_1.*dtheta_2.*t3.*t8.*t22.*t23.*2.0+I_b.*dtheta_1.*dtheta_2.*t8.*t14.*t18.*t20.*4.0-I_b.*dtheta_1.*dtheta_2.*t8.*t14.*t19.*t20-I_b.*dtheta_1.*dtheta_2.*t8.*t14.*t20.*t22-I_b.*d2theta_1.*r_b.*t3.*t4.*t5.*t14+I_b.*d2theta_1.*r_b.*t4.*t5.*t14.*t16+I_b.*d2theta_2.*r_b.*t2.*t3.*t20.*t22+I_b.*d2theta_1.*t3.*t4.*t6.*t15.*t22-I_b.*d2theta_1.*t3.*t5.*t8.*t14.*t20+I_b.*d2theta_2.*t3.*t4.*t8.*t15.*t22+I_b.*d2theta_2.*t2.*t3.*t8.*t21.*t22+I_b.*d2theta_1.*t5.*t8.*t14.*t16.*t20-I_b.*d2theta_2.*t5.*t6.*t14.*t18.*t20-I_b.*d2theta_2.*t3.*t6.*t14.*t20.*t24+I_b.*dtheta_1.*t3.*t4.*t7.*t15.*t22-I_b.*dtheta_1.*t3.*t5.*t9.*t14.*t20+I_b.*dtheta_2.*t3.*t4.*t9.*t15.*t22.*2.0+I_b.*dtheta_2.*t2.*t3.*t9.*t21.*t22.*2.0+I_b.*dtheta_1.*t5.*t9.*t14.*t16.*t20.*2.0-I_b.*dtheta_2.*t5.*t7.*t14.*t18.*t20.*2.0-I_b.*dtheta_2.*t3.*t7.*t14.*t20.*t24.*2.0+I_b.*r_b.*t2.*t5.*t10.*t16.*t20+I_b.*r_b.*t2.*t5.*t11.*t16.*t20.*2.0-I_b.*t3.*t4.*t5.*t8.*t10.*t15+I_b.*t4.*t5.*t8.*t10.*t15.*t16+I_b.*t4.*t5.*t8.*t11.*t15.*t16.*2.0+I_b.*t4.*t5.*t8.*t10.*t15.*t18+I_b.*t2.*t5.*t8.*t10.*t16.*t21+I_b.*t2.*t5.*t8.*t11.*t16.*t21.*2.0-I_b.*t3.*t6.*t10.*t14.*t20.*t22-I_b.*t6.*t11.*t14.*t16.*t20.*t22.*3.0+dtheta_1.*dtheta_2.*m_b.*t4.*t13.*t14.*t22-dtheta_1.*dtheta_2.*t4.*t6.*t15.*t24.*t28+dtheta_1.*dtheta_2.*t3.*t8.*t17.*t22.*t28.*2.0+dtheta_1.*dtheta_2.*t8.*t14.*t20.*t22.*t28+d2theta_1.*m_b.*t4.*t5.*t13.*t14.*t16+d2theta_2.*t3.*t4.*t8.*t15.*t22.*t28+d2theta_1.*t5.*t8.*t14.*t16.*t20.*t28-dtheta_1.*t3.*t4.*t7.*t15.*t22.*t28+dtheta_1.*t3.*t5.*t9.*t14.*t20.*t28+dtheta_2.*t3.*t4.*t9.*t15.*t22.*t28.*2.0+dtheta_1.*t5.*t9.*t14.*t16.*t20.*t28.*2.0+m_b.*t2.*t3.*t5.*t10.*t13.*t20.*2.0+m_b.*t2.*t5.*t10.*t13.*t16.*t20+t3.*t4.*t5.*t8.*t10.*t15.*t28+t2.*t3.*t5.*t8.*t10.*t21.*t28.*2.0+t4.*t5.*t8.*t10.*t15.*t16.*t28+t4.*t5.*t8.*t11.*t15.*t16.*t28+t4.*t5.*t8.*t10.*t15.*t18.*t28+t2.*t5.*t8.*t10.*t16.*t21.*t28-t3.*t6.*t10.*t14.*t20.*t22.*t28+I_b.*dtheta_1.*dtheta_2.*r_b.*t3.*t4.*t14.*t22.*2.0+I_b.*dtheta_1.*dtheta_2.*t4.*t5.*t6.*t15.*t16+I_b.*dtheta_1.*dtheta_2.*t3.*t8.*t14.*t20.*t22.*4.0-I_b.*dtheta_1.*dtheta_2.*t8.*t14.*t16.*t20.*t22+dtheta_1.*dtheta_2.*m_b.*t3.*t4.*t13.*t14.*t22.*2.0+dtheta_1.*dtheta_2.*t3.*t8.*t14.*t20.*t22.*t28.*2.0))./(t16+t22);t9;-t26.*t27.*t31.*t32.*(I_b.*d2theta_1.*r_b.*t3.*t15+I_b.*r_b.*t10.*t16.*t21.*2.0+I_b.*t3.*t8.*t10.*t17+I_b.*t8.*t10.*t16.*t17-I_b.*t8.*t10.*t17.*t18+I_b.*t8.*t10.*t16.*t23.*2.0+d2z_C.*t4.*t15.*t18.*t28+g.*t4.*t15.*t18.*t28+m_b.*t10.*t13.*t16.*t21.*2.0-t3.*t8.*t10.*t17.*t28+t8.*t10.*t16.*t17.*t28.*2.0-t8.*t10.*t17.*t18.*t28+t8.*t10.*t16.*t23.*t28.*2.0+d2theta_1.*m_b.*t2.*t13.*t16.*t20+d2theta_1.*t4.*t8.*t15.*t16.*t28-d2theta_2.*t4.*t6.*t15.*t18.*t28+d2theta_1.*t2.*t8.*t16.*t21.*t28-dtheta_1.*t3.*t4.*t9.*t15.*t28+dtheta_1.*t3.*t5.*t7.*t17.*t28+dtheta_1.*t4.*t9.*t15.*t16.*t28.*2.0-dtheta_2.*t4.*t7.*t15.*t18.*t28.*2.0+dtheta_1.*t4.*t9.*t15.*t18.*t28+dtheta_1.*t2.*t9.*t16.*t21.*t28.*2.0-m_b.*t3.*t4.*t10.*t13.*t14.*2.0+m_b.*t4.*t10.*t13.*t14.*t16.*3.0+m_b.*t4.*t11.*t13.*t14.*t16+m_b.*t4.*t11.*t13.*t14.*t22.*2.0-t3.*t8.*t10.*t14.*t20.*t28.*2.0-t4.*t6.*t11.*t15.*t24.*t28.*2.0+t8.*t10.*t14.*t16.*t20.*t28.*4.0+t8.*t11.*t14.*t16.*t20.*t28+t8.*t11.*t14.*t20.*t22.*t28.*2.0+I_b.*dtheta_1.*dtheta_2.*r_b.*t5.*t15-I_b.*dtheta_1.*dtheta_2.*t6.*t16.*t17-I_b.*dtheta_1.*dtheta_2.*t6.*t17.*t22+I_b.*d2theta_1.*r_b.*t2.*t16.*t20+I_b.*d2theta_1.*t3.*t4.*t8.*t15-I_b.*d2theta_1.*t3.*t5.*t6.*t17+I_b.*d2theta_1.*t4.*t8.*t15.*t16-I_b.*d2theta_1.*t4.*t8.*t15.*t18+I_b.*d2theta_1.*t2.*t8.*t16.*t21+I_b.*dtheta_1.*t3.*t4.*t9.*t15-I_b.*dtheta_1.*t3.*t5.*t7.*t17+I_b.*dtheta_1.*t4.*t9.*t15.*t16.*2.0-I_b.*dtheta_1.*t4.*t9.*t15.*t18+I_b.*dtheta_1.*t2.*t9.*t16.*t21.*2.0+I_b.*r_b.*t4.*t10.*t14.*t16.*2.0+I_b.*t8.*t10.*t14.*t16.*t20.*3.0-dtheta_1.*dtheta_2.*m_b.*t5.*t13.*t15+dtheta_1.*dtheta_2.*t6.*t17.*t22.*t28+I_b.*dtheta_1.*dtheta_2.*t4.*t5.*t8.*t15+I_b.*t3.*t4.*t5.*t6.*t10.*t15-dtheta_1.*dtheta_2.*t4.*t5.*t8.*t15.*t28+d2theta_2.*m_b.*t3.*t4.*t5.*t13.*t14-d2theta_2.*t3.*t4.*t6.*t15.*t22.*t28+d2theta_2.*t3.*t5.*t8.*t14.*t20.*t28-dtheta_2.*t3.*t4.*t7.*t15.*t22.*t28.*2.0+dtheta_2.*t3.*t5.*t9.*t14.*t20.*t28.*2.0+t3.*t4.*t5.*t6.*t10.*t15.*t28-t4.*t5.*t6.*t10.*t15.*t16.*t28-t4.*t5.*t6.*t11.*t15.*t16.*t28.*2.0+I_b.*dtheta_1.*dtheta_2.*t4.*t5.*t8.*t15.*t16+dtheta_1.*dtheta_2.*m_b.*t2.*t3.*t5.*t13.*t20.*2.0+dtheta_1.*dtheta_2.*t3.*t4.*t5.*t8.*t15.*t28.*2.0+dtheta_1.*dtheta_2.*t2.*t3.*t5.*t8.*t21.*t28.*2.0)];
end

== matlab function BallAndPlateSimulation/Simulate sensors/MATLAB Function ==
  data: theta1 input; P_A output; theta2 input; theta3 input; Zc input; P_B output; P_C output
% Roll-Pitch-Yaw angles to motors position
% Roll (theta1): rotation about x-axis
% Pitch (theta2): rotation about y-axis
% Yaw (theta3): rotation about z-axis
% See page 12 and Appendix A (Multibody and Nonlinear Dynamics lecture
% notes for further reference
% Motors (1,2,3) -> (A,B,C)

function [P_A, P_B, P_C] = anglesToMotors(theta1,theta2,theta3,Zc)

%% Define parameters
r = 0.17;
r0B1 = [r; 0; 0];      
r0B2 = [-0.5*r; (sqrt(3)/2)*r; 0];
r0B3 = [-0.5*r; -(sqrt(3)/2)*r; 0];
r0B = [r0B1 r0B2 r0B3];
%r1C1 = r0B1; r1C2 = r0B2; r1C3 = r0B3;
r1C = r0B;
r0Oc = [0;0;Zc];

% Find cos and sin to accelerate calculations
C1 = cos(theta1);S1 = sin(theta1);C2 = cos(theta2);S2 = sin(theta2);C3 = cos(theta3);S3 = sin(theta3);

% Rotation matrices
RotZ = [C3 S3 0; -S3 C3 0; 0 0 1];
RotY = [C2 0 -S2; 0 1 0; S2 0 C2];
RotX = [1 0 0; 0 C1 S1; 0 -S1 C1];

A10 = RotX*RotY*RotZ; A01 = A10';

% Find rCiBi (Vectors representing the motors)
rCiBi = zeros(3,3);
for i=1:3
    rCiBi(:,i) = r0Oc + A01*r1C(:,i) - r0B(:,i);
end

% Outputs to motor are the lengths of the vectors
P_A = norm(rCiBi(:,1));
P_B = norm(rCiBi(:,2));
P_C = norm(rCiBi(:,3));
end
